simulink model "StateSpace"  (R2021a)
settings: Solver=FixedStepAuto  StartTime=0.0  StopTime=STime  FixedStep=1e-3  RelTol=1e-3
undefined symbols (not defined in the file): C, J, K_, Kp, Mc, Ra, Ta, Tp, TPert
settings Model: Creator=akangmufti  LastModifiedBy=akangmufti
settings OptimizationCC: DefaultParameterBehavior=Inlined  BufferReuse=off
settings DebuggingCC: InitInArrayFormatMsg=none

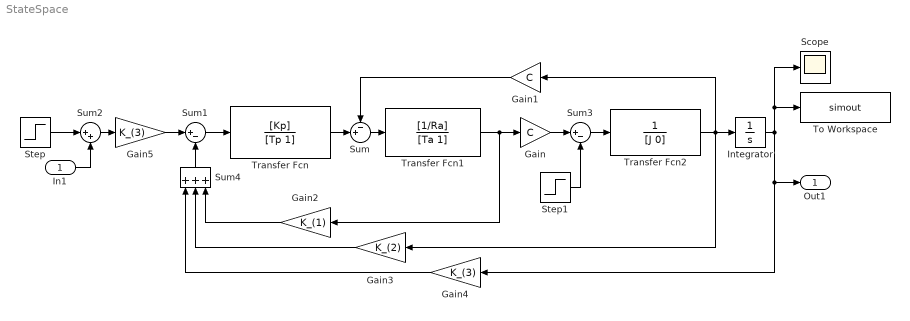
== system StateSpace ==
  In1 : Inport
  Gain : Gain  Gain=C
  Gain1 : Gain  Gain=C
  Gain2 : Gain  Gain=K_(1)
  Gain3 : Gain  Gain=K_(2)
  Gain4 : Gain  Gain=K_(3)
  Gain5 : Gain  Gain=K_(3)
  Integrator : Integrator
  Scope : Scope
  Step : Step  Time=1e-3  SampleTime=0
  Step1 : Step  Time=TPert  After=Mc  SampleTime=0
  Sum : Sum  Inputs=-+|
  Sum1 : Sum  Inputs=|+-
  Sum2 : Sum  Inputs=|++
  Sum3 : Sum  Inputs=|+-
  Sum4 : Sum  Inputs=+++
  To Workspace : ToWorkspace  VariableName=simout  SampleTime=-1
  Transfer Fcn : TransferFcn  Numerator=[Kp]  Denominator=[Tp 1]
  Transfer Fcn1 : TransferFcn  Numerator=[1/Ra]  Denominator=[Ta 1]
  Transfer Fcn2 : TransferFcn  Denominator=[J 0]
  Out1 : Outport
  wires:
  In1/1 -> Sum2/2
  Gain/1 -> Sum3/1
  Sum/1 -> Transfer Fcn1/1
  Transfer Fcn1/1 -> Gain2/1, Gain/1
  Transfer Fcn/1 -> Sum/2
  Gain1/1 -> Sum/1
  Sum3/1 -> Transfer Fcn2/1
  Transfer Fcn2/1 -> Gain3/1, Integrator/1, Gain1/1
  Step1/1 -> Sum3/2
  Gain3/1 -> Sum4/2
  Gain4/1 -> Sum4/1
  Gain2/1 -> Sum4/3
  Sum4/1 -> Sum1/2
  Sum1/1 -> Transfer Fcn/1
  Sum2/1 -> Gain5/1
  Gain5/1 -> Sum1/1
  Integrator/1 -> Scope/1, To Workspace/1, Gain4/1, Out1/1
  Step/1 -> Sum2/1
